simulink model "generic"  (Simulink 10.0)
settings: Solver=ode45  StartTime=0.0  StopTime=inf  RelTol=1e-3  EnableMultiTasking=on
libraries: CarMaker4SL x64, simulink x6
(part 2 of 3)

== system generic/CarMaker/IPG Vehicle/CarAndTrailer/Forces/Vehicle Forces ==
  Sync_In : Inport
  Bus Creator1 : BusCreator  Inputs=12
  Bus Creator8 : BusCreator  Inputs=16
  BusCreator1 : BusCreator  Inputs=4
  BusCreator2 : BusCreator  Inputs=9
  Demux : Demux  Outputs=16
  Demux1 : Demux  Outputs=12
  Demux2 : Demux  Outputs=13
  Forces : S-Function  FunctionName=CM_Sfun  Parameters='Forces'  SFunctionDeploymentMode=off  EnableBusSupport=off
  Terminator : Terminator
  Sync_Out : Outport
  Car.Virtual : Outport  Port=2
  Car.Aero : Outport  Port=3
  Car.Load : Outport  Port=4
  wires:
  BusCreator1/1 -> Terminator/1  "Aero IF (in)"
  Demux2/13 -> BusCreator2/9  "car Aero Trq_1 z"
  Demux2/12 -> BusCreator2/8  "car Aero Trq_1 y"
  Demux2/11 -> BusCreator2/7  "car Aero Trq_1 x"
  Demux2/10 -> BusCreator2/6  "car Aero Frc_1 z"
  Demux2/9 -> BusCreator2/5  "car Aero Frc_1 y"
  Demux2/8 -> BusCreator2/4  "car Aero Frc_1 x"
  Demux2/7 -> BusCreator2/3  "car Aero PoA_1 z"
  Demux2/6 -> BusCreator2/2  "car Aero PoA_1 y"
  Demux2/5 -> BusCreator2/1  "car Aero PoA_1 x"
  Demux2/4 -> BusCreator1/4  "car Aero tau_1"
  Demux2/3 -> BusCreator1/3  "car Aero ApproachVel_1 z"
  Demux2/2 -> BusCreator1/2  "car Aero ApproachVel_1 y"
  Demux2/1 -> BusCreator1/1  "car Aero ApproachVel_1 x"
  Demux/16 -> Bus Creator8/16  "Car Load_3 tz"
  Demux/15 -> Bus Creator8/15  "Car Load_3 ty"
  Demux/14 -> Bus Creator8/14  "Car Load_3 tx"
  Demux/13 -> Bus Creator8/13  "Car Load_3 mass"
  Demux1/12 -> Bus Creator1/12  "Car Virtual Trq_0 z"
  Demux1/11 -> Bus Creator1/11  "Car Virtual Trq_0 y"
  Demux1/10 -> Bus Creator1/10  "Car Virtual Trq_0 x"
  Demux1/9 -> Bus Creator1/9  "Car Virtual Trq_1 z"
  Demux1/8 -> Bus Creator1/8  "Car Virtual Trq_1 y"
  Demux1/7 -> Bus Creator1/7  "Car Virtual Trq_1 x"
  Demux1/6 -> Bus Creator1/6  "Car Virtual Frc_0 z"
  Demux1/5 -> Bus Creator1/5  "Car Virtual Frc_0 y"
  Demux1/4 -> Bus Creator1/4  "Car Virtual Frc_0 x"
  Sync_In/1 -> Forces/1
  Forces/1 -> Sync_Out/1
  BusCreator2/1 -> Car.Aero/1
  Demux1/1 -> Bus Creator1/1  "Car Virtual Frc_1 x"
  Demux1/2 -> Bus Creator1/2  "Car Virtual Frc_1 y"
  Demux1/3 -> Bus Creator1/3  "Car Virtual Frc_1 z"
  Forces/3 -> Demux2/1
  Forces/2 -> Demux1/1
  Bus Creator1/1 -> Car.Virtual/1
  Bus Creator8/1 -> Car.Load/1
  Demux/1 -> Bus Creator8/1  "Car Load_0 mass"
  Demux/2 -> Bus Creator8/2  "Car Load_0 tx"
  Demux/3 -> Bus Creator8/3  "Car Load_0 ty"
  Demux/4 -> Bus Creator8/4  "Car Load_0 tz"
  Demux/5 -> Bus Creator8/5  "Car Load_1 mass"
  Demux/6 -> Bus Creator8/6  "Car Load_1 tx"
  Demux/7 -> Bus Creator8/7  "Car Load_1 ty"
  Demux/8 -> Bus Creator8/8  "Car Load_1 tz"
  Demux/9 -> Bus Creator8/9  "Car Load_2 mass"
  Demux/10 -> Bus Creator8/10  "Car Load_2 tx"
  Demux/11 -> Bus Creator8/11  "Car Load_2 ty"
  Demux/12 -> Bus Creator8/12  "Car Load_2 tz"
  Forces/4 -> Demux/1

== system generic/CarMaker/IPG Vehicle/CarAndTrailer/Trailer/CreateBus Car.Hitch.FrcTrq ==
  In1 : Inport
  Bus Creator7 : BusCreator  Inputs=6
  Demux7 : Demux  Outputs=6
  Out1 : Outport
  wires:
  In1/1 -> Demux7/1
  Bus Creator7/1 -> Out1/1
  Demux7/6 -> Bus Creator7/6  "Car Hitch Trq2Car z"
  Demux7/5 -> Bus Creator7/5  "Car Hitch Trq2Car y"
  Demux7/4 -> Bus Creator7/4  "Car Hitch Trq2Car x"
  Demux7/3 -> Bus Creator7/3  "Car Hitch Frc2Car z"
  Demux7/2 -> Bus Creator7/2  "Car Hitch Frc2Car y"
  Demux7/1 -> Bus Creator7/1  "Car Hitch Frc2Car x"

== system generic/CarMaker/IPG Vehicle/CarAndTrailer/Trailer/CreateBus Vhcl.Motion ==
  In1 : Inport
  BusCreator : BusCreator  Inputs=15
  Demux : Demux  Outputs=15
  Out1 : Outport
  wires:
  Demux/15 -> BusCreator/15  "Vhcl YawAcc"
  Demux/14 -> BusCreator/14  "Vhcl YawVel"
  Demux/13 -> BusCreator/13  "Vhcl Yaw"
  Demux/12 -> BusCreator/12  "Vhcl PitchAcc"
  Demux/11 -> BusCreator/11  "Vhcl PitchVel"
  Demux/10 -> BusCreator/10  "Vhcl Pitch"
  Demux/9 -> BusCreator/9  "Vhcl RollAcc"
  Demux/8 -> BusCreator/8  "Vhcl RollVel"
  Demux/7 -> BusCreator/7  "Vhcl Roll"
  Demux/6 -> BusCreator/6  "Vhcl Hitch_Pos z"
  Demux/5 -> BusCreator/5  "Vhcl Hitch_Pos y"
  Demux/4 -> BusCreator/4  "Vhcl Hitch_Pos x"
  Demux/3 -> BusCreator/3  "Vhcl sRoad"
  Demux/2 -> BusCreator/2  "Vhcl Distance"
  Demux/1 -> BusCreator/1  "Vhcl v"
  In1/1 -> Demux/1
  BusCreator/1 -> Out1/1

== system generic/CarMaker/IPG Vehicle/CarAndTrailer/Trailer/CreateBus Vhcl.PoI ==
  In1 : Inport
  Bus Creator3 : BusCreator  Inputs=18
  Demux3 : Demux  Outputs=18
  Out1 : Outport
  wires:
  Demux3/18 -> Bus Creator3/18  "Vhcl PoI_GCS Elev"
  Demux3/17 -> Bus Creator3/17  "Vhcl PoI_GCS Lat"
  Demux3/16 -> Bus Creator3/16  "Vhcl PoI_GCS Long"
  Demux3/15 -> Bus Creator3/15  "Vhcl PoI_Acc_1 z"
  Demux3/14 -> Bus Creator3/14  "Vhcl PoI_Acc_1 y"
  Demux3/13 -> Bus Creator3/13  "Vhcl PoI_Acc_1 x"
  Demux3/12 -> Bus Creator3/12  "Vhcl PoI_Vel_1 z"
  Demux3/11 -> Bus Creator3/11  "Vhcl PoI_Vel_1 y"
  Demux3/10 -> Bus Creator3/10  "Vhcl PoI_Vel_1 x"
  Demux3/9 -> Bus Creator3/9  "Vhcl PoI_Acc z"
  Demux3/8 -> Bus Creator3/8  "Vhcl PoI_Acc y"
  Demux3/7 -> Bus Creator3/7  "Vhcl PoI_Acc x"
  Demux3/6 -> Bus Creator3/6  "Vhcl PoI_Vel z"
  Demux3/5 -> Bus Creator3/5  "Vhcl PoI_Vel y"
  Demux3/4 -> Bus Creator3/4  "Vhcl PoI_Vel x"
  Demux3/3 -> Bus Creator3/3  "Vhcl PoI_Pos z"
  Demux3/2 -> Bus Creator3/2  "Vhcl PoI_Pos y"
  In1/1 -> Demux3/1
  Bus Creator3/1 -> Out1/1
  Demux3/1 -> Bus Creator3/1  "Vhcl PoI_Pos x"

== system generic/CarMaker/IPG Vehicle/CarAndTrailer/Trailer/CreateBus Vhcl.Steering ==
  In1 : Inport
  Bus Creator3 : BusCreator  Inputs=4
  Demux : Demux
  Out1 : Outport
  wires:
  Bus Creator3/1 -> Out1/1
  Demux/1 -> Bus Creator3/1  "Vhcl Steering Ang"
  Demux/3 -> Bus Creator3/3  "Vhcl Steering AngAcc"
  Demux/2 -> Bus Creator3/2  "Vhcl Steering AngVel"
  Demux/4 -> Bus Creator3/4  "Vhcl Steering Trq"
  In1/1 -> Demux/1

== system generic/CarMaker/IPG Vehicle/CarAndTrailer/Trailer/CreateBus Vhcl.Wheel.FL ==
  In1 : Inport
  Bus Creator3 : BusCreator  Inputs=14
  Demux3 : Demux  Outputs=14
  Out1 : Outport
  wires:
  Demux3/14 -> Bus Creator3/14  "Vhcl Wheel FL Trq_WhlBearing"
  Demux3/13 -> Bus Creator3/13  "Vhcl Wheel FL Trq_T2W"
  Demux3/12 -> Bus Creator3/12  "Vhcl Wheel FL SideSlip"
  Demux3/11 -> Bus Creator3/11  "Vhcl Wheel FL LongSlip"
  Demux3/10 -> Bus Creator3/10  "Vhcl Wheel FL vBelt"
  Demux3/9 -> Bus Creator3/9  "Vhcl Wheel FL Fz"
  Demux3/8 -> Bus Creator3/8  "Vhcl Wheel FL Fy"
  Demux3/7 -> Bus Creator3/7  "Vhcl Wheel FL Fx"
  Demux3/6 -> Bus Creator3/6  "Vhcl Wheel FL r_zxy z"
  Demux3/5 -> Bus Creator3/5  "Vhcl Wheel FL r_zxy y"
  Demux3/4 -> Bus Creator3/4  "Vhcl Wheel FL r_zxy x"
  Demux3/3 -> Bus Creator3/3  "Vhcl Wheel FL t z"
  Demux3/2 -> Bus Creator3/2  "Vhcl Wheel FL t y"
  In1/1 -> Demux3/1
  Bus Creator3/1 -> Out1/1
  Demux3/1 -> Bus Creator3/1  "Vhcl Wheel FL t x"

== system generic/CarMaker/IPG Vehicle/CarAndTrailer/Trailer/CreateBus Vhcl.Wheel.FR ==
  In1 : Inport
  Bus Creator3 : BusCreator  Inputs=14
  Demux3 : Demux  Outputs=14
  Out1 : Outport
  wires:
  Demux3/14 -> Bus Creator3/14  "Vhcl Wheel FR Trq_WhlBearing"
  Demux3/13 -> Bus Creator3/13  "Vhcl Wheel FR Trq_T2W"
  Demux3/12 -> Bus Creator3/12  "Vhcl Wheel FR SideSlip"
  Demux3/11 -> Bus Creator3/11  "Vhcl Wheel FR LongSlip"
  Demux3/10 -> Bus Creator3/10  "Vhcl Wheel FR vBelt"
  Demux3/9 -> Bus Creator3/9  "Vhcl Wheel FR Fz"
  Demux3/8 -> Bus Creator3/8  "Vhcl Wheel FR Fy"
  Demux3/7 -> Bus Creator3/7  "Vhcl Wheel FR Fx"
  Demux3/6 -> Bus Creator3/6  "Vhcl Wheel FR r_zxy z"
  Demux3/5 -> Bus Creator3/5  "Vhcl Wheel FR r_zxy y"
  Demux3/4 -> Bus Creator3/4  "Vhcl Wheel FR r_zxy x"
  Demux3/3 -> Bus Creator3/3  "Vhcl Wheel FR t z"
  Demux3/2 -> Bus Creator3/2  "Vhcl Wheel FR t y"
  In1/1 -> Demux3/1
  Bus Creator3/1 -> Out1/1
  Demux3/1 -> Bus Creator3/1  "Vhcl Wheel FR t x"

== system generic/CarMaker/IPG Vehicle/CarAndTrailer/Trailer/CreateBus Vhcl.Wheel.RL ==
  In1 : Inport
  Bus Creator3 : BusCreator  Inputs=14
  Demux3 : Demux  Outputs=14
  Out1 : Outport
  wires:
  Demux3/14 -> Bus Creator3/14  "Vhcl Wheel RL Trq_WhlBearing"
  Demux3/13 -> Bus Creator3/13  "Vhcl Wheel RL Trq_T2W"
  Demux3/12 -> Bus Creator3/12  "Vhcl Wheel RL SideSlip"
  Demux3/11 -> Bus Creator3/11  "Vhcl Wheel RL LongSlip"
  Demux3/10 -> Bus Creator3/10  "Vhcl Wheel RL vBelt"
  Demux3/9 -> Bus Creator3/9  "Vhcl Wheel RL Fz"
  Demux3/8 -> Bus Creator3/8  "Vhcl Wheel RL Fy"
  Demux3/7 -> Bus Creator3/7  "Vhcl Wheel RL Fx"
  Demux3/6 -> Bus Creator3/6  "Vhcl Wheel RL r_zxy z"
  Demux3/5 -> Bus Creator3/5  "Vhcl Wheel RL r_zxy y"
  Demux3/4 -> Bus Creator3/4  "Vhcl Wheel RL r_zxy x"
  Demux3/3 -> Bus Creator3/3  "Vhcl Wheel RL t z"
  Demux3/2 -> Bus Creator3/2  "Vhcl Wheel RL t y"
  In1/1 -> Demux3/1
  Bus Creator3/1 -> Out1/1
  Demux3/1 -> Bus Creator3/1  "Vhcl Wheel RL t x"

== system generic/CarMaker/IPG Vehicle/CarAndTrailer/Trailer/CreateBus Vhcl.Wheel.RR ==
  In1 : Inport
  Bus Creator3 : BusCreator  Inputs=14
  Demux3 : Demux  Outputs=14
  Out1 : Outport
  wires:
  Demux3/14 -> Bus Creator3/14  "Vhcl Wheel RR Trq_WhlBearing"
  Demux3/13 -> Bus Creator3/13  "Vhcl Wheel RR Trq_T2W"
  Demux3/12 -> Bus Creator3/12  "Vhcl Wheel RR SideSlip"
  Demux3/11 -> Bus Creator3/11  "Vhcl Wheel RR LongSlip"
  Demux3/10 -> Bus Creator3/10  "Vhcl Wheel RR vBelt"
  Demux3/9 -> Bus Creator3/9  "Vhcl Wheel RR Fz"
  Demux3/8 -> Bus Creator3/8  "Vhcl Wheel RR Fy"
  Demux3/7 -> Bus Creator3/7  "Vhcl Wheel RR Fx"
  Demux3/6 -> Bus Creator3/6  "Vhcl Wheel RR r_zxy z"
  Demux3/5 -> Bus Creator3/5  "Vhcl Wheel RR r_zxy y"
  Demux3/4 -> Bus Creator3/4  "Vhcl Wheel RR r_zxy x"
  Demux3/3 -> Bus Creator3/3  "Vhcl Wheel RR t z"
  Demux3/2 -> Bus Creator3/2  "Vhcl Wheel RR t y"
  In1/1 -> Demux3/1
  Bus Creator3/1 -> Out1/1
  Demux3/1 -> Bus Creator3/1  "Vhcl Wheel RR t x"

== system generic/CarMaker/VehicleControl/CreateBus VhclCtrl/Braking/Front Camera ==
  Bus Selector : BusSelector  OutputSignals=MBR_TR_X,MBR_BL_Y,MBR_TR_Y,Confidence
  Camera Sensor Object : CarMaker4SL/Sensors/Camera Sensor Object  xname=Frontcamera  xstime=Inherited
      settings: SourceProductName=CarMaker4SL
  Constant1 : Constant
  Constant7 : Constant
  Data Type Conversion : DataTypeConversion  OutDataTypeStr=double
  Ground5 : Ground
  If : If  NumInputs=4  IfExpression=(u1>0&u3<0) &u4>0  ElseIfExpressions=((u1<=0.55&u1>=-0.55)|(u3<=0.55&u3>=-0.55))&u4>0,u2==0&u4>0  ShowElse=off
  If Action Subsystem : Subsystem  TreatAsAtomicUnit=on
  If Action Subsystem1 : Subsystem  TreatAsAtomicUnit=on
  If Action Subsystem2 : Subsystem  TreatAsAtomicUnit=on
  Terminator : Terminator
  While Iterator Subsystem3 : Subsystem  TreatAsAtomicUnit=on
  wires:
  Constant7/1 -> While Iterator Subsystem3/1(IC)
  Bus Selector/2 -> If Action Subsystem2/2(Inport1), If/1  "<MBR_BL_Y>"
  Bus Selector/3 -> If Action Subsystem2/3(Inport2), If/3  "<MBR_TR_Y>"
  Bus Selector/1 -> If Action Subsystem2/1(Inport), If Action Subsystem/1(Inport), If/2  "<MBR_TR_X>"
  If/3 -> If Action Subsystem1/Action
  Data Type Conversion/1 -> If/4
  If/1 -> If Action Subsystem/Action
  Camera Sensor Object/1 -> Terminator/1
  Ground5/1 -> Camera Sensor Object/1
  Constant1/1 -> Camera Sensor Object/2
  Camera Sensor Object/2 -> Bus Selector/1
  Bus Selector/4 -> Data Type Conversion/1  "<Confidence>"
  If/2 -> If Action Subsystem2/Action

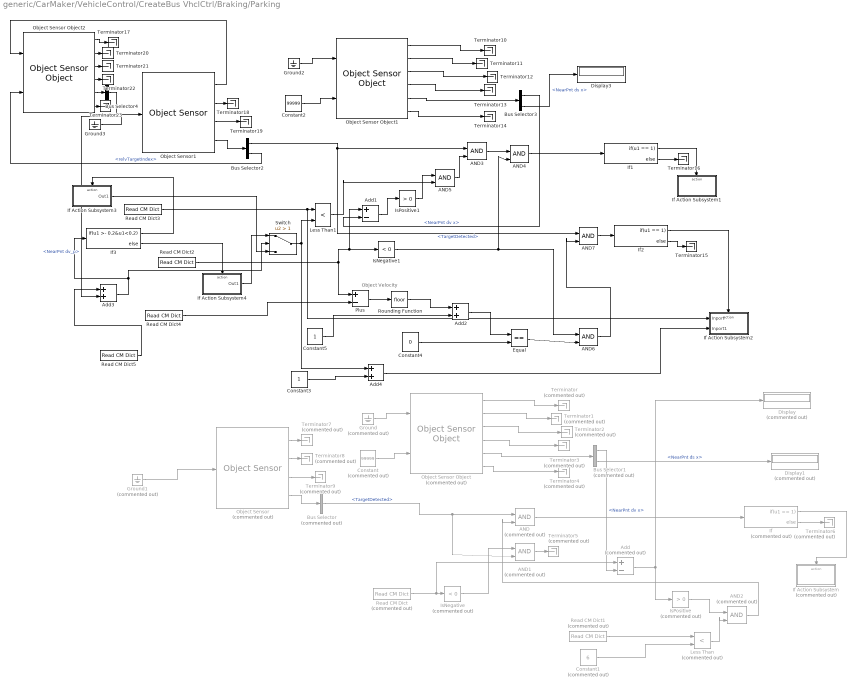
== system generic/CarMaker/VehicleControl/CreateBus VhclCtrl/Braking/Parking ==
  note: Object Velocity
  AND : Logic  Commented=on  IconShape=distinctive  AllPortsSameDT=off  OutDataTypeStr=boolean
  AND1 : Logic  Commented=on  IconShape=distinctive  AllPortsSameDT=off  OutDataTypeStr=boolean
  AND2 : Logic  Commented=on  IconShape=distinctive  AllPortsSameDT=off  OutDataTypeStr=boolean
  AND{3..7} (5 alike) : Logic  IconShape=distinctive  AllPortsSameDT=off  OutDataTypeStr=boolean
  Add : Sum  Commented=on  Inputs=+-
  Add1 : Sum  Inputs=+-
  Add2 : Sum
  Add3 : Sum
  Add4 : Sum
  Bus Selector : BusSelector  Commented=on  OutputSignals=TargetDetected
  Bus Selector1 : BusSelector  Commented=on  OutputSignals=NearPnt dv x,NearPnt ds x
  Bus Selector2 : BusSelector  OutputSignals=TargetDetected,relvTargetIndex
  Bus Selector3 : BusSelector  OutputSignals=NearPnt dv x,NearPnt ds x
  Bus Selector4 : BusSelector  OutputSignals=NearPnt dv_p
  Constant : Constant  Commented=on  Value=99999
  Constant1 : Constant  Commented=on  Value=6
  Constant2 : Constant  Value=99999
  Constant3 : Constant
  Constant4 : Constant  Value=0
  Constant5 : Constant
  Display : Display  Commented=on
  Display1 : Display  Commented=on
  Display3 : Display
  Equal : RelationalOperator  Operator===  OutDataTypeStr=boolean  RndMeth=Simplest
  Ground : Ground  Commented=on
  Ground1 : Ground  Commented=on
  Ground2 : Ground
  Ground3 : Ground
  If : If  Commented=on  IfExpression=u1 == 1
  If Action Subsystem : Subsystem  Commented=on  TreatAsAtomicUnit=on
  If Action Subsystem1 : Subsystem  TreatAsAtomicUnit=on
  If Action Subsystem2 : Subsystem  TreatAsAtomicUnit=on
  If Action Subsystem3 : Subsystem  TreatAsAtomicUnit=on
  If Action Subsystem4 : Subsystem  TreatAsAtomicUnit=on
  If1 : If  IfExpression=u1 == 1
  If2 : If  IfExpression=u1 == 1
  If3 : If  IfExpression=u1 >- 0.2&u1<0.2
  IsNegative : simulink/Logic and Bit Operations/Compare To Zero  Commented=on  relop=<  OutDataTypeStr=boolean
  IsNegative1 : simulink/Logic and Bit Operations/Compare To Zero  relop=<  OutDataTypeStr=boolean
  IsPositive : simulink/Logic and Bit Operations/Compare To Zero  Commented=on  relop=>  OutDataTypeStr=boolean
  IsPositive1 : simulink/Logic and Bit Operations/Compare To Zero  relop=>  OutDataTypeStr=boolean
  Less Than : RelationalOperator  Commented=on  Operator=<  OutDataTypeStr=boolean  RndMeth=Simplest
  Less Than1 : RelationalOperator  Operator=<  OutDataTypeStr=boolean  RndMeth=Simplest
  Object Sensor : CarMaker4SL/Sensors/Object Sensor  Commented=on  xname=RearR  xstime=Continuous
      settings: SourceProductName=CarMaker4SL
  Object Sensor Object : CarMaker4SL/Sensors/Object Sensor Object  Commented=on  xname=RearR  ximode=Observed Objects  xstime=Continuous
      settings: SourceProductName=CarMaker4SL
  Object Sensor Object1 : CarMaker4SL/Sensors/Object Sensor Object  xname=RearC  ximode=Observed Objects  xstime=Continuous
      settings: SourceProductName=CarMaker4SL
  Object Sensor Object2 : CarMaker4SL/Sensors/Object Sensor Object  xname=INPORT  ximode=Observed Objects  xstime=Continuous
      settings: SourceProductName=CarMaker4SL
  Object Sensor1 : CarMaker4SL/Sensors/Object Sensor  xname=RearC  xstime=Continuous
      settings: SourceProductName=CarMaker4SL
  Plus : Sum  Inputs=+-
  Read CM Dict : CarMaker4SL/Read CM Dict  Commented=on  xname=Car.vx  xsync=off  xstime=Continuous
  Read CM Dict1 : CarMaker4SL/Read CM Dict  Commented=on  xname=Sensor.Object.RearR.relvTgt.NearPnt.ds.x  xsync=off  xstime=Continuous
  Read CM Dict2 : CarMaker4SL/Read CM Dict  xname=Car.vx  xsync=off  xstime=Continuous
  Read CM Dict3 : CarMaker4SL/Read CM Dict  xname=Sensor.Object.RearC.relvTgt.NearPnt.ds.x  xsync=off  xstime=Continuous
  Read CM Dict4 : CarMaker4SL/Read CM Dict  xname=Sensor.Object.RearC.relvTgt.RefPnt.dv_p  xsync=off  xstime=Continuous
  Read CM Dict5 : CarMaker4SL/Read CM Dict  xname=Car.v  xsync=off  xstime=Continuous
  Rounding Function : Rounding
  Switch : Switch  Criteria=u2 > Threshold  Threshold=1
  Terminator{,1..9} (10 alike) : Terminator  Commented=on
  Terminator{10..23} (14 alike) : Terminator
  wires:
  Bus Selector3/2 -> Display3/1  "<NearPnt ds x>"
  Bus Selector2/1 -> AND3/1, AND7/1  "<TargetDetected>"
  Object Sensor Object1/1 -> Terminator10/1
  AND5/1 -> AND3/2
  Ground2/1 -> Object Sensor Object1/1
  Constant2/1 -> Object Sensor Object1/2
  Object Sensor Object1/2 -> Terminator11/1
  Object Sensor Object1/6 -> Terminator14/1
  IsPositive1/1 -> AND5/1
  Add1/1 -> IsPositive1/1
  Object Sensor Object1/4 -> Terminator13/1
  Object Sensor1/1 -> Object Sensor Object2/1
  Read CM Dict3/1 -> If Action Subsystem2/1(Inport), Less Than1/1
  Less Than1/1 -> AND5/2
  Object Sensor1/4 -> Bus Selector2/1
  If1/2 -> Terminator16/1
  Object Sensor Object1/3 -> Terminator12/1
  Object Sensor Object1/5 -> Bus Selector3/1
  Read CM Dict2/1 -> Add1/1, IsNegative1/1, Plus/1
  Bus Selector3/1 -> Add1/2  "<NearPnt dv x>"
  If1/1 -> If Action Subsystem1/Action
  Object Sensor1/2 -> Terminator18/1
  Ground3/1 -> Object Sensor1/1
  Object Sensor1/3 -> Terminator19/1
  Read CM Dict4/1 -> Plus/2
  Constant4/1 -> Equal/2
  Plus/1 -> Rounding Function/1
  Equal/1 -> AND6/2
  AND4/1 -> If1/1
  AND3/1 -> AND4/1
  IsNegative1/1 -> AND6/1, AND4/2
  Rounding Function/1 -> Add2/1
  Constant5/1 -> Add2/2
  Add2/1 -> Equal/1
  AND6/1 -> AND7/2
  AND7/1 -> If2/1
  If2/1 -> If Action Subsystem2/Action
  If2/2 -> Terminator15/1
  If/1 -> If Action Subsystem/Action
  Ground1/1 -> Object Sensor/1
  IsPositive/1 -> AND2/1
  AND/1 -> If/1
  Bus Selector1/2 -> Display1/1  "<NearPnt ds x>"
  Object Sensor/2 -> Terminator8/1
  AND2/1 -> AND/2
  Add/1 -> IsPositive/1, Display/1
  Bus Selector1/1 -> Add/2  "<NearPnt dv x>"
  Object Sensor Object/6 -> Terminator4/1
  If/2 -> Terminator6/1
  Less Than/1 -> AND2/2
  Object Sensor Object/4 -> Terminator3/1
  Constant/1 -> Object Sensor Object/2
  AND1/1 -> Terminator5/1
  Read CM Dict1/1 -> Less Than/1
  Object Sensor Object/5 -> Bus Selector1/1
  Object Sensor Object/1 -> Terminator/1
  Object Sensor/1 -> Terminator7/1
  Object Sensor/3 -> Terminator9/1
  Object Sensor Object/2 -> Terminator1/1
  Constant1/1 -> Less Than/2
  IsNegative/1 -> AND1/1
  Object Sensor Object/3 -> Terminator2/1
  Read CM Dict/1 -> Add/1, IsNegative/1
  Bus Selector/1 -> AND1/2, AND/1  "<TargetDetected>"
  Ground/1 -> Object Sensor Object/1
  Object Sensor/4 -> Bus Selector/1
  Read CM Dict5/1 -> Add3/1
  If3/1 -> If Action Subsystem3/Action
  Bus Selector2/2 -> Object Sensor Object2/2  "<relvTargetIndex>"
  Object Sensor Object2/1 -> Terminator17/1
  Object Sensor Object2/2 -> Terminator20/1
  Object Sensor Object2/3 -> Terminator21/1
  Object Sensor Object2/4 -> Terminator22/1
  Object Sensor Object2/5 -> Bus Selector4/1
  Object Sensor Object2/6 -> Terminator23/1
  Bus Selector4/1 -> Add3/2  "<NearPnt dv_p>"
  If3/2 -> If Action Subsystem4/Action
  Switch/1 -> Less Than1/2, Add4/1
  Add3/1 -> Switch/2, If3/1
  Add4/1 -> If Action Subsystem2/2(Inport1)
  Constant3/1 -> Add4/2
  If Action Subsystem4/1(Out1) -> Switch/1
  If Action Subsystem3/1(Out1) -> Switch/3

== system generic/CarMaker/VehicleControl/CreateBus VhclCtrl/Braking/Short ==
  Bus Selector : BusSelector  OutputSignals=TargetDetected
  Ground1 : Ground
  If Action Subsystem1 : Subsystem  TreatAsAtomicUnit=on
  If1 : If  IfExpression=u1 == 1
  Object Sensor : CarMaker4SL/Sensors/Object Sensor  xname=UltrasonicFront  xstime=Continuous
      settings: SourceProductName=CarMaker4SL
  Read CM Dict : CarMaker4SL/Read CM Dict  xname=Sensor.Object.UltrasonicFront.relvTgt.NearPnt.ds.x  xsync=off  xstime=Continuous
  Read CM Dict1 : CarMaker4SL/Read CM Dict  xname=Sensor.Object.UltrasonicFront.relvTgt.NearPnt.dv_p  xsync=off  xstime=Continuous
  Terminator{,2..4} (4 alike) : Terminator
  wires:
  Object Sensor/4 -> Bus Selector/1
  If1/1 -> If Action Subsystem1/Action
  Object Sensor/2 -> Terminator2/1
  If1/2 -> Terminator/1
  Read CM Dict/1 -> If Action Subsystem1/1(In1)
  Object Sensor/1 -> Terminator3/1
  Ground1/1 -> Object Sensor/1
  Read CM Dict1/1 -> If Action Subsystem1/2(In2)
  Bus Selector/1 -> If1/1  "<TargetDetected>"
  Object Sensor/3 -> Terminator4/1

== system generic/CarMaker/VehicleControl/CreateBus VhclCtrl/Braking/Subsystem6 ==
  Bus Selector1 : BusSelector  OutputSignals=nObj
  Constant1 : Constant
  Ground : Ground
  Radar Sensor : CarMaker4SL/Sensors/Radar Sensor  xname=RoadDetection  xstime=Continuous
      settings: SourceProductName=CarMaker4SL
  Terminator2 : Terminator
  While Iterator Subsystem : Subsystem  TreatAsAtomicUnit=on
  wires:
  Constant1/1 -> While Iterator Subsystem/2(Inport)
  Radar Sensor/1 -> Terminator2/1
  Bus Selector1/1 -> While Iterator Subsystem/1(Input)  "<nObj>"
  Radar Sensor/2 -> Bus Selector1/1
  Ground/1 -> Radar Sensor/1

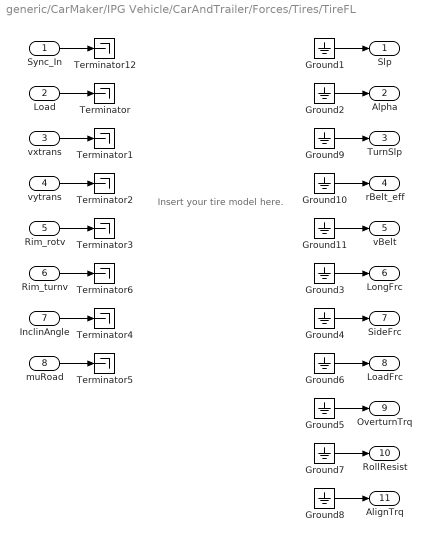
== system generic/CarMaker/IPG Vehicle/CarAndTrailer/Forces/Tires/TireFL ==
  note: Insert your tire model here.
  Sync_In : Inport
  Load : Inport  Port=2
  vxtrans : Inport  Port=3
  vytrans : Inport  Port=4
  Rim_rotv : Inport  Port=5
  Rim_turnv : Inport  Port=6
  InclinAngle : Inport  Port=7
  muRoad : Inport  Port=8
  Ground{1..11} (11 alike) : Ground
  Terminator{,1..6,12} (8 alike) : Terminator
  Slp : Outport
  Alpha : Outport  Port=2
  TurnSlp : Outport  Port=3
  rBelt_eff : Outport  Port=4
  vBelt : Outport  Port=5
  LongFrc : Outport  Port=6
  SideFrc : Outport  Port=7
  LoadFrc : Outport  Port=8
  OverturnTrq : Outport  Port=9
  RollResist : Outport  Port=10
  AlignTrq : Outport  Port=11
  wires:
  Ground11/1 -> vBelt/1
  Ground10/1 -> rBelt_eff/1
  Ground9/1 -> TurnSlp/1
  Rim_turnv/1 -> Terminator6/1
  Sync_In/1 -> Terminator12/1
  Ground2/1 -> Alpha/1
  Ground3/1 -> LongFrc/1
  Ground4/1 -> SideFrc/1
  Ground5/1 -> OverturnTrq/1
  vxtrans/1 -> Terminator1/1
  vytrans/1 -> Terminator2/1
  Rim_rotv/1 -> Terminator3/1
  InclinAngle/1 -> Terminator4/1
  muRoad/1 -> Terminator5/1
  Load/1 -> Terminator/1
  Ground1/1 -> Slp/1
  Ground6/1 -> LoadFrc/1
  Ground7/1 -> RollResist/1
  Ground8/1 -> AlignTrq/1

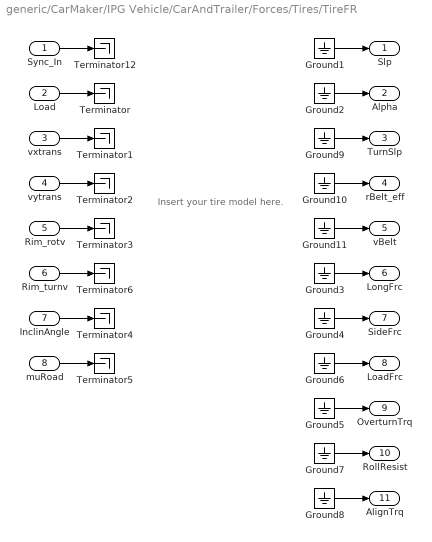
== system generic/CarMaker/IPG Vehicle/CarAndTrailer/Forces/Tires/TireFR ==
  note: Insert your tire model here.
  Sync_In : Inport
  Load : Inport  Port=2
  vxtrans : Inport  Port=3
  vytrans : Inport  Port=4
  Rim_rotv : Inport  Port=5
  Rim_turnv : Inport  Port=6
  InclinAngle : Inport  Port=7
  muRoad : Inport  Port=8
  Ground{1..11} (11 alike) : Ground
  Terminator{,1..6,12} (8 alike) : Terminator
  Slp : Outport
  Alpha : Outport  Port=2
  TurnSlp : Outport  Port=3
  rBelt_eff : Outport  Port=4
  vBelt : Outport  Port=5
  LongFrc : Outport  Port=6
  SideFrc : Outport  Port=7
  LoadFrc : Outport  Port=8
  OverturnTrq : Outport  Port=9
  RollResist : Outport  Port=10
  AlignTrq : Outport  Port=11
  wires:
  Ground11/1 -> vBelt/1
  Ground10/1 -> rBelt_eff/1
  Ground9/1 -> TurnSlp/1
  Rim_turnv/1 -> Terminator6/1
  Sync_In/1 -> Terminator12/1
  Ground2/1 -> Alpha/1
  Ground3/1 -> LongFrc/1
  Ground4/1 -> SideFrc/1
  Ground5/1 -> OverturnTrq/1
  vxtrans/1 -> Terminator1/1
  vytrans/1 -> Terminator2/1
  Rim_rotv/1 -> Terminator3/1
  InclinAngle/1 -> Terminator4/1
  muRoad/1 -> Terminator5/1
  Load/1 -> Terminator/1
  Ground1/1 -> Slp/1
  Ground6/1 -> LoadFrc/1
  Ground7/1 -> RollResist/1
  Ground8/1 -> AlignTrq/1

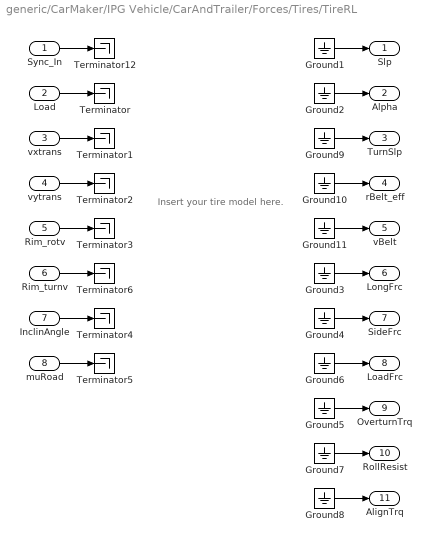
== system generic/CarMaker/IPG Vehicle/CarAndTrailer/Forces/Tires/TireRL ==
  note: Insert your tire model here.
  Sync_In : Inport
  Load : Inport  Port=2
  vxtrans : Inport  Port=3
  vytrans : Inport  Port=4
  Rim_rotv : Inport  Port=5
  Rim_turnv : Inport  Port=6
  InclinAngle : Inport  Port=7
  muRoad : Inport  Port=8
  Ground{1..11} (11 alike) : Ground
  Terminator{,1..6,12} (8 alike) : Terminator
  Slp : Outport
  Alpha : Outport  Port=2
  TurnSlp : Outport  Port=3
  rBelt_eff : Outport  Port=4
  vBelt : Outport  Port=5
  LongFrc : Outport  Port=6
  SideFrc : Outport  Port=7
  LoadFrc : Outport  Port=8
  OverturnTrq : Outport  Port=9
  RollResist : Outport  Port=10
  AlignTrq : Outport  Port=11
  wires:
  Ground11/1 -> vBelt/1
  Ground10/1 -> rBelt_eff/1
  Ground9/1 -> TurnSlp/1
  Rim_turnv/1 -> Terminator6/1
  Sync_In/1 -> Terminator12/1
  Ground2/1 -> Alpha/1
  Ground3/1 -> LongFrc/1
  Ground4/1 -> SideFrc/1
  Ground5/1 -> OverturnTrq/1
  vxtrans/1 -> Terminator1/1
  vytrans/1 -> Terminator2/1
  Rim_rotv/1 -> Terminator3/1
  InclinAngle/1 -> Terminator4/1
  muRoad/1 -> Terminator5/1
  Load/1 -> Terminator/1
  Ground1/1 -> Slp/1
  Ground6/1 -> LoadFrc/1
  Ground7/1 -> RollResist/1
  Ground8/1 -> AlignTrq/1

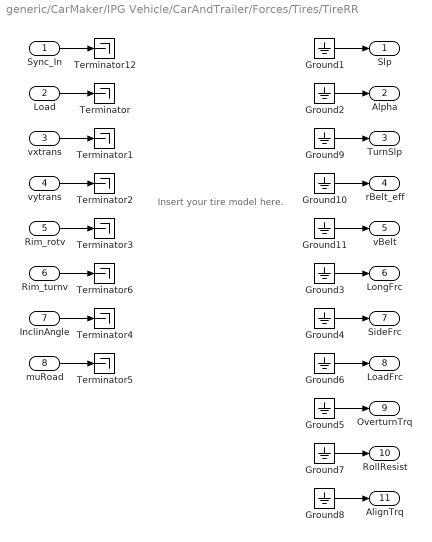
== system generic/CarMaker/IPG Vehicle/CarAndTrailer/Forces/Tires/TireRR ==
  note: Insert your tire model here.
  Sync_In : Inport
  Load : Inport  Port=2
  vxtrans : Inport  Port=3
  vytrans : Inport  Port=4
  Rim_rotv : Inport  Port=5
  Rim_turnv : Inport  Port=6
  InclinAngle : Inport  Port=7
  muRoad : Inport  Port=8
  Ground{1..11} (11 alike) : Ground
  Terminator{,1..6,12} (8 alike) : Terminator
  Slp : Outport
  Alpha : Outport  Port=2
  TurnSlp : Outport  Port=3
  rBelt_eff : Outport  Port=4
  vBelt : Outport  Port=5
  LongFrc : Outport  Port=6
  SideFrc : Outport  Port=7
  LoadFrc : Outport  Port=8
  OverturnTrq : Outport  Port=9
  RollResist : Outport  Port=10
  AlignTrq : Outport  Port=11
  wires:
  Ground11/1 -> vBelt/1
  Ground10/1 -> rBelt_eff/1
  Ground9/1 -> TurnSlp/1
  Rim_turnv/1 -> Terminator6/1
  Sync_In/1 -> Terminator12/1
  Ground2/1 -> Alpha/1
  Ground3/1 -> LongFrc/1
  Ground4/1 -> SideFrc/1
  Ground5/1 -> OverturnTrq/1
  vxtrans/1 -> Terminator1/1
  vytrans/1 -> Terminator2/1
  Rim_rotv/1 -> Terminator3/1
  InclinAngle/1 -> Terminator4/1
  muRoad/1 -> Terminator5/1
  Load/1 -> Terminator/1
  Ground1/1 -> Slp/1
  Ground6/1 -> LoadFrc/1
  Ground7/1 -> RollResist/1
  Ground8/1 -> AlignTrq/1

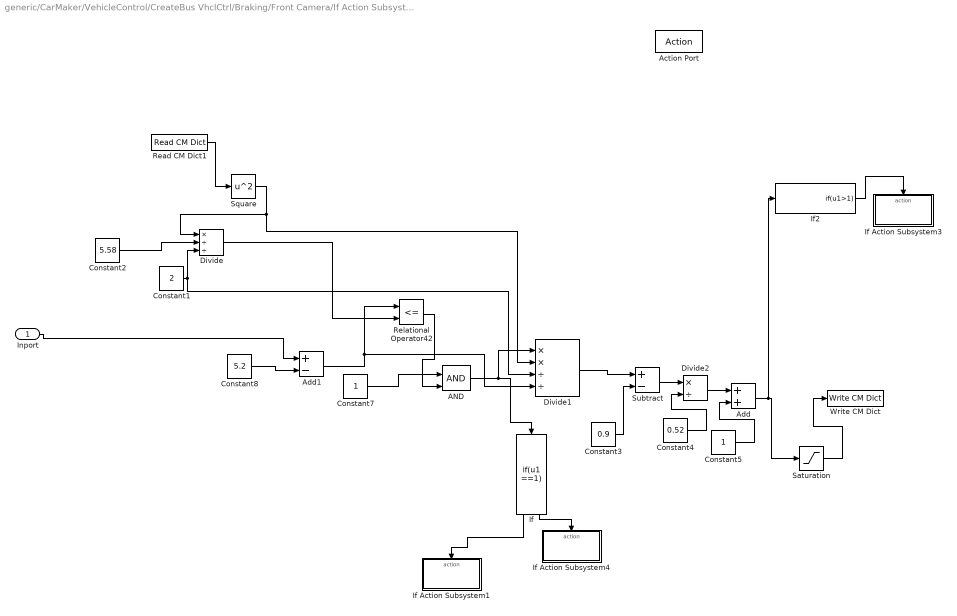
== system generic/CarMaker/VehicleControl/CreateBus VhclCtrl/Braking/Front Camera/If Action Subsystem ==
  Inport : Inport
  Action Port : ActionPort  ActionPortLabel=if((u1>0&u3<0) &u4>0)
  AND : Logic  IconShape=distinctive  AllPortsSameDT=off  OutDataTypeStr=boolean
  Add : Sum
  Add1 : Sum  Inputs=+-
  Constant1 : Constant  Value=2
  Constant2 : Constant  Value=5.58
  Constant3 : Constant  Value=0.9
  Constant4 : Constant  Value=0.52
  Constant5 : Constant
  Constant7 : Constant
  Constant8 : Constant  Value=5.2
  Divide : Product  Inputs=*//
  Divide1 : Product  Inputs=**//
  Divide2 : Product  Inputs=*/
  If : If  IfExpression=u1 ==1
  If Action Subsystem1 : Subsystem  TreatAsAtomicUnit=on
  If Action Subsystem3 : Subsystem  TreatAsAtomicUnit=on
  If Action Subsystem4 : Subsystem  TreatAsAtomicUnit=on
  If2 : If  IfExpression=u1>1  ShowElse=off
  Read CM Dict1 : CarMaker4SL/Read CM Dict  xname=Car.vx  xsync=off  xstime=Inherited
  Relational Operator42 : RelationalOperator  Operator=<=  OutDataTypeStr=boolean  RndMeth=Simplest
  Saturation : Saturate  UpperLimit=1  LowerLimit=0
  Square : Math  Operator=square  SaturateOnIntegerOverflow=on
  Subtract : Sum  Inputs=+-
  Write CM Dict : CarMaker4SL/Write CM Dict  xname=VC.Brake  xsync=off
  wires:
  AND/1 -> If/1, Divide1/1
  If/2 -> If Action Subsystem4/Action
  Subtract/1 -> Divide2/1
  Add1/1 -> Divide1/4, Relational Operator42/1
  Square/1 -> Divide1/2, Divide/1
  Saturation/1 -> Write CM Dict/1
  Constant4/1 -> Divide2/2
  Constant7/1 -> AND/1
  Constant5/1 -> Add/2
  Constant2/1 -> Divide/2
  Constant8/1 -> Add1/2
  Constant3/1 -> Subtract/2
  Divide1/1 -> Subtract/1
  If/1 -> If Action Subsystem1/Action
  Constant1/1 -> Divide/3, Divide1/3
  Inport/1 -> Add1/1
  Divide2/1 -> Add/1
  Read CM Dict1/1 -> Square/1
  Divide/1 -> Relational Operator42/2
  Relational Operator42/1 -> AND/2
  Add/1 -> If2/1, Saturation/1
  If2/1 -> If Action Subsystem3/Action

== system generic/CarMaker/VehicleControl/CreateBus VhclCtrl/Braking/Front Camera/If Action Subsystem1 ==
  Action Port : ActionPort  ActionPortLabel=elseif(u2==0&u4>0)
  Constant : Constant
  Constant1 : Constant
  Write CM Dict : CarMaker4SL/Write CM Dict  xname=VC.Brake  xsync=off
  Write CM Dict1 : CarMaker4SL/Write CM Dict  xname=VC.Gas  xsync=off
  wires:
  Constant/1 -> Write CM Dict/1
  Constant1/1 -> Write CM Dict1/1

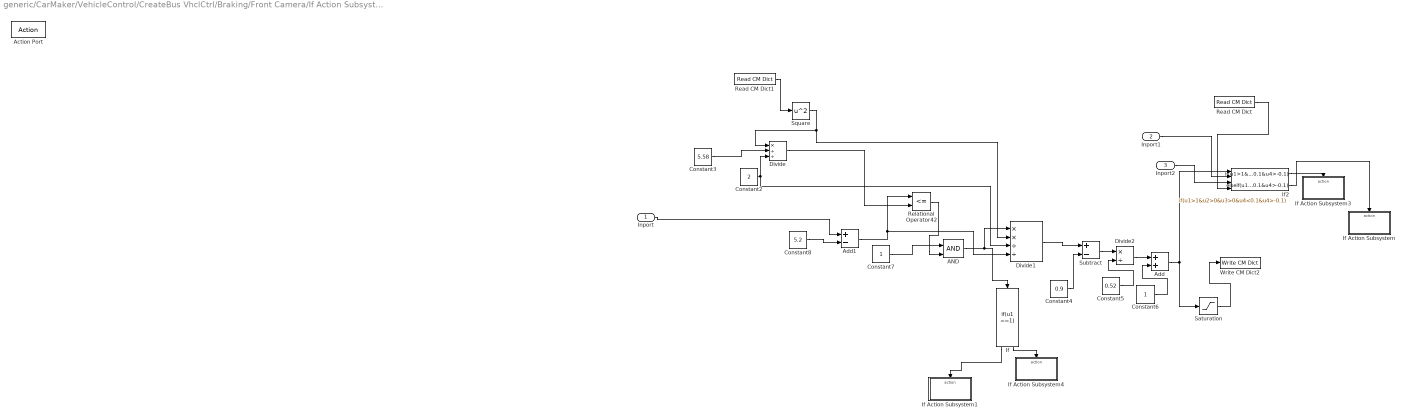
== system generic/CarMaker/VehicleControl/CreateBus VhclCtrl/Braking/Front Camera/If Action Subsystem2 ==
  Inport : Inport
  Inport1 : Inport  Port=2
  Inport2 : Inport  Port=3
  Action Port : ActionPort  ActionPortLabel=elseif(((u1<=0.55&u1>=-0.55)|(u3<=0.55&u3>=-0.55))&u4>0)
  AND : Logic  IconShape=distinctive  AllPortsSameDT=off  OutDataTypeStr=boolean
  Add : Sum
  Add1 : Sum  Inputs=+-
  Constant2 : Constant  Value=2
  Constant3 : Constant  Value=5.58
  Constant4 : Constant  Value=0.9
  Constant5 : Constant  Value=0.52
  Constant6 : Constant
  Constant7 : Constant
  Constant8 : Constant  Value=5.2
  Divide : Product  Inputs=*//
  Divide1 : Product  Inputs=**//
  Divide2 : Product  Inputs=*/
  If : If  IfExpression=u1 ==1
  If Action Subsystem : Subsystem  TreatAsAtomicUnit=on
  If Action Subsystem1 : Subsystem  TreatAsAtomicUnit=on
  If Action Subsystem3 : Subsystem  TreatAsAtomicUnit=on
  If Action Subsystem4 : Subsystem  TreatAsAtomicUnit=on
  If2 : If  NumInputs=4  IfExpression=u1>1&u2>0&u3>0&u4<0.1&u4>-0.1  ElseIfExpressions=u1>1&u2<0&u3<0&u4<0.1&u4>-0.1  ShowElse=off
  Read CM Dict : CarMaker4SL/Read CM Dict  xname=DM.Steer.Ang  xsync=off  xstime=Inherited
  Read CM Dict1 : CarMaker4SL/Read CM Dict  xname=Car.vx  xsync=off  xstime=Inherited
  Relational Operator42 : RelationalOperator  Operator=<=  OutDataTypeStr=boolean  RndMeth=Simplest
  Saturation : Saturate  UpperLimit=1  LowerLimit=0
  Square : Math  Operator=square  SaturateOnIntegerOverflow=on
  Subtract : Sum  Inputs=+-
  Write CM Dict2 : CarMaker4SL/Write CM Dict  xname=VC.Brake  xsync=off
  wires:
  Subtract/1 -> Divide2/1
  Divide/1 -> Relational Operator42/2
  Relational Operator42/1 -> AND/2
  Constant8/1 -> Add1/2
  Read CM Dict1/1 -> Square/1
  Saturation/1 -> Write CM Dict2/1
  Square/1 -> Divide1/2, Divide/1
  Divide2/1 -> Add/1
  Inport/1 -> Add1/1
  Constant5/1 -> Divide2/2
  Constant7/1 -> AND/1
  Constant2/1 -> Divide/3, Divide1/3
  Constant3/1 -> Divide/2
  If/1 -> If Action Subsystem1/Action
  Divide1/1 -> Subtract/1
  AND/1 -> If/1, Divide1/1
  Constant6/1 -> Add/2
  Add1/1 -> Divide1/4, Relational Operator42/1
  Constant4/1 -> Subtract/2
  If/2 -> If Action Subsystem4/Action
  Read CM Dict/1 -> If2/4
  Add/1 -> If2/1, Saturation/1
  If2/2 -> If Action Subsystem/Action
  If2/1 -> If Action Subsystem3/Action
  Inport1/1 -> If2/2
  Inport2/1 -> If2/3

== system generic/CarMaker/VehicleControl/CreateBus VhclCtrl/Braking/Front Camera/While Iterator Subsystem3 ==
  IC : Inport
  Bus Selector : BusSelector  OutputSignals=MBR_TR_X,MBR_BL_Y,MBR_TR_Y,Confidence
  Camera Sensor Object : CarMaker4SL/Sensors/Camera Sensor Object  xname=Frontcamera  xstime=Inherited
      settings: SourceProductName=CarMaker4SL
  Constant : Constant
  Constant1 : Constant
  Constant2 : Constant  Value=0
  Data Type Conversion : DataTypeConversion  OutDataTypeStr=double
  Ground5 : Ground
  If : If  NumInputs=4  IfExpression=(u1>0&u3<0) &u4>0  ElseIfExpressions=((u1<=0.55&u1>=-0.55)|(u3<=0.55&u3>=-0.55))&u4>0,u2==0&u4>0  ShowElse=off
  If Action Subsystem : Subsystem  TreatAsAtomicUnit=on
  If Action Subsystem1 : Subsystem  TreatAsAtomicUnit=on
  If Action Subsystem2 : Subsystem  TreatAsAtomicUnit=on
  Subtract : Sum  Inputs=+-
  Terminator : Terminator
  While Iterator : WhileIterator  MaxIters=4  ShowIterationPort=on
  wires:
  IC/1 -> While Iterator/2
  Ground5/1 -> Camera Sensor Object/1
  Camera Sensor Object/2 -> Bus Selector/1
  Camera Sensor Object/1 -> Terminator/1
  If/1 -> If Action Subsystem/Action
  Bus Selector/1 -> If Action Subsystem2/1(Inport), If Action Subsystem/1(Inport), If/2  "<MBR_TR_X>"
  Constant1/1 -> Subtract/2
  Constant/1 -> While Iterator/1
  Bus Selector/4 -> Data Type Conversion/1  "<Confidence>"
  Data Type Conversion/1 -> If/4
  If/2 -> If Action Subsystem2/Action
  Bus Selector/2 -> If/1  "<MBR_BL_Y>"
  Bus Selector/3 -> If/3  "<MBR_TR_Y>"
  While Iterator/1 -> Subtract/1
  If/3 -> If Action Subsystem1/Action
  Constant2/1 -> Camera Sensor Object/2

== system generic/CarMaker/VehicleControl/CreateBus VhclCtrl/Braking/Parking/If Action Subsystem ==
  Action Port : ActionPort
  Constant : Constant  Value=0
  Constant1 : Constant
  Write CM Dict : CarMaker4SL/Write CM Dict  xname=VC.Gas  xsync=off
  Write CM Dict1 : CarMaker4SL/Write CM Dict  xname=VC.Brake  xsync=off
  wires:
  Constant/1 -> Write CM Dict/1
  Constant1/1 -> Write CM Dict1/1

== system generic/CarMaker/VehicleControl/CreateBus VhclCtrl/Braking/Parking/If Action Subsystem1 ==
  Action Port : ActionPort  ActionPortLabel=if(u1 == 1)
  Constant : Constant  Value=0
  Constant1 : Constant
  Write CM Dict : CarMaker4SL/Write CM Dict  xname=VC.Gas  xsync=off
  Write CM Dict1 : CarMaker4SL/Write CM Dict  xname=VC.Brake  xsync=off
  wires:
  Constant/1 -> Write CM Dict/1
  Constant1/1 -> Write CM Dict1/1

== system generic/CarMaker/VehicleControl/CreateBus VhclCtrl/Braking/Parking/If Action Subsystem2 ==
  Inport : Inport
  Inport1 : Inport  Port=2
  Action Port : ActionPort  ActionPortLabel=if(u1 == 1)
  Constant1 : Constant  Value=1.4
  If : If  NumInputs=2  IfExpression=u1 ==1 &u2~=1  ElseIfExpressions=u2==1 &u1==1
  If Action Subsystem : Subsystem  TreatAsAtomicUnit=on
  If Action Subsystem1 : Subsystem  TreatAsAtomicUnit=on
  Less Than : RelationalOperator  Operator=<  OutDataTypeStr=boolean  RndMeth=Simplest
  Less Than1 : RelationalOperator  Operator=<  OutDataTypeStr=boolean  RndMeth=Simplest
  Terminator : Terminator
  wires:
  Inport/1 -> Less Than1/1, Less Than/1
  Inport1/1 -> Less Than/2
  Less Than/1 -> If/1
  If/3 -> Terminator/1
  If/1 -> If Action Subsystem/Action
  Constant1/1 -> Less Than1/2
  If/2 -> If Action Subsystem1/Action
  Less Than1/1 -> If/2

== system generic/CarMaker/VehicleControl/CreateBus VhclCtrl/Braking/Parking/If Action Subsystem3 ==
  Action Port : ActionPort  ActionPortLabel=if(u1 >- 0.2&u1<0.2)
  Constant : Constant
  Out1 : Outport
  wires:
  Constant/1 -> Out1/1

== system generic/CarMaker/VehicleControl/CreateBus VhclCtrl/Braking/Parking/If Action Subsystem4 ==
  Action Port : ActionPort  ActionPortLabel=else
  Constant : Constant  Value=5
  Out1 : Outport
  wires:
  Constant/1 -> Out1/1

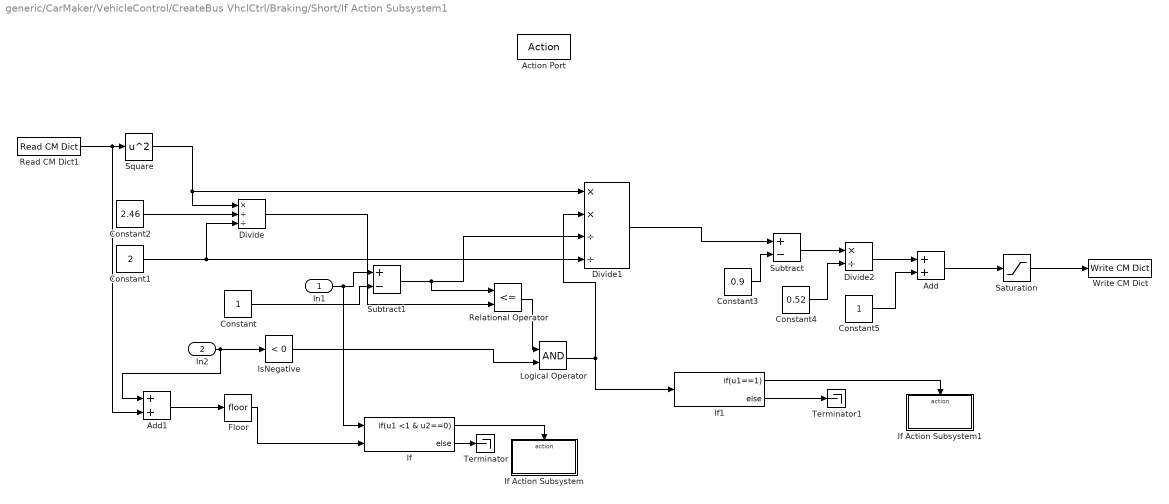
== system generic/CarMaker/VehicleControl/CreateBus VhclCtrl/Braking/Short/If Action Subsystem1 ==
  In1 : Inport
  In2 : Inport  Port=2
  Action Port : ActionPort  ActionPortLabel=if(u1 == 1)
  Add : Sum
  Add1 : Sum
  Constant : Constant
  Constant1 : Constant  Value=2
  Constant2 : Constant  Value=2.46  VectorParams1D=off
  Constant3 : Constant  Value=0.9
  Constant4 : Constant  Value=0.52
  Constant5 : Constant
  Divide : Product  Inputs=*//
  Divide1 : Product  Inputs=**//
  Divide2 : Product  Inputs=*/
  Floor : Rounding
  If : If  NumInputs=2  IfExpression=u1 <1 & u2==0
  If Action Subsystem : Subsystem  TreatAsAtomicUnit=on
  If Action Subsystem1 : Subsystem  TreatAsAtomicUnit=on
  If1 : If  IfExpression=u1==1
  IsNegative : simulink/Logic and Bit Operations/Compare To Zero  relop=<  OutDataTypeStr=boolean
  Logical Operator : Logic  AllPortsSameDT=off  OutDataTypeStr=boolean
  Read CM Dict1 : CarMaker4SL/Read CM Dict  xname=Car.vx  xsync=off  xstime=Continuous
  Relational Operator : RelationalOperator  Operator=<=  OutDataTypeStr=boolean  RndMeth=Simplest
  Saturation : Saturate  UpperLimit=1  LowerLimit=0
  Square : Math  Operator=square  SaturateOnIntegerOverflow=on
  Subtract : Sum  Inputs=+-
  Subtract1 : Sum  Inputs=+-
  Terminator : Terminator
  Terminator1 : Terminator
  Write CM Dict : CarMaker4SL/Write CM Dict  xname=VC.Brake  xsync=off
  wires:
  Add/1 -> Saturation/1
  Constant3/1 -> Subtract/2
  Relational Operator/1 -> Logical Operator/1
  IsNegative/1 -> Logical Operator/2
  Divide2/1 -> Add/1
  Divide1/1 -> Subtract/1
  Subtract/1 -> Divide2/1
  Read CM Dict1/1 -> Add1/2, Square/1
  Constant1/1 -> Divide/3, Divide1/4
  Constant4/1 -> Divide2/2
  Logical Operator/1 -> Divide1/2, If1/1
  In1/1 -> If/1, Subtract1/1
  If1/2 -> Terminator1/1
  Divide/1 -> Relational Operator/2
  Saturation/1 -> Write CM Dict/1
  Square/1 -> Divide1/1, Divide/1
  Constant2/1 -> Divide/2
  Constant5/1 -> Add/2
  If1/1 -> If Action Subsystem1/Action
  In2/1 -> Add1/1, IsNegative/1
  Constant/1 -> Subtract1/2
  Subtract1/1 -> Relational Operator/1, Divide1/3
  If/2 -> Terminator/1
  If/1 -> If Action Subsystem/Action
  Add1/1 -> Floor/1
  Floor/1 -> If/2

== system generic/CarMaker/VehicleControl/CreateBus VhclCtrl/Braking/Subsystem6/While Iterator Subsystem ==
  Input : Inport
  Inport : Inport  Port=2
  Bus Selector : BusSelector  OutputSignals=DistY,DistX,VrelX,DistZ
  Constant1 : Constant
  Ground1 : Ground
  If : If  NumInputs=4  IfExpression=u1<0.4&u1>-0.4&u4~=0&u3<0.3&u3>-0.3&u1<1  ShowElse=off
  If Action Subsystem1 : Subsystem  TreatAsAtomicUnit=on
  Radar Sensor Object : CarMaker4SL/Sensors/Radar Sensor Object  xname=RoadDetection  ximode=Observed Objects  xstime=Inherited
      settings: SourceProductName=CarMaker4SL
  Read CM Dict1 : CarMaker4SL/Read CM Dict  xname=Car.vx  xsync=off  xstime=Inherited
  Relational Operator : RelationalOperator  OutDataTypeStr=boolean  RndMeth=Simplest
  Subtract : Sum  Inputs=+-
  Terminator : Terminator
  VxO : Sum
  While Iterator : WhileIterator  MaxIters=100  ResetStates=reset  ShowIterationPort=on
  wires:
  Inport/1 -> While Iterator/2
  Ground1/1 -> Radar Sensor Object/1
  Radar Sensor Object/1 -> Terminator/1
  While Iterator/1 -> Relational Operator/2, Subtract/1
  Bus Selector/1 -> If/1  "<DistY>"
  Radar Sensor Object/2 -> Bus Selector/1
  Subtract/1 -> Radar Sensor Object/2
  Bus Selector/2 -> If Action Subsystem1/1(Inport), If/2  "<DistX>"
  Constant1/1 -> Subtract/2
  Read CM Dict1/1 -> VxO/1
  VxO/1 -> If/3
  Input/1 -> Relational Operator/1
  Relational Operator/1 -> While Iterator/1
  If/1 -> If Action Subsystem1/Action
  Bus Selector/3 -> VxO/2  "<VrelX>"
  Bus Selector/4 -> If/4  "<DistZ>"

== system generic/CarMaker/VehicleControl/CreateBus VhclCtrl/Braking/Front Camera/If Action Subsystem/If Action Subsystem1 ==
  Action Port : ActionPort  ActionPortLabel=if(u1 ==1)
  Constant : Constant  Value=0
  Write CM Dict1 : CarMaker4SL/Write CM Dict  xname=VC.Gas  xsync=off
  wires:
  Constant/1 -> Write CM Dict1/1

== system generic/CarMaker/VehicleControl/CreateBus VhclCtrl/Braking/Front Camera/If Action Subsystem/If Action Subsystem3 ==
  Action Port : ActionPort  ActionPortLabel=if(u1>1)
  Constant : Constant  Commented=on  Value=30
  Constant1 : Constant  Commented=on  Value=-3
  Write CM Dict : CarMaker4SL/Write CM Dict  Commented=on  xname=VC.Steer.AngAcc  xsync=off
  Write CM Dict1 : CarMaker4SL/Write CM Dict  Commented=on  xname=VC.Steer.Ang  xsync=off
  wires:
  Constant/1 -> Write CM Dict/1
  Constant1/1 -> Write CM Dict1/1

== system generic/CarMaker/VehicleControl/CreateBus VhclCtrl/Braking/Front Camera/If Action Subsystem/If Action Subsystem4 ==
  Action Port : ActionPort  ActionPortLabel=else

== system generic/CarMaker/VehicleControl/CreateBus VhclCtrl/Braking/Front Camera/If Action Subsystem2/If Action Subsystem ==
  Action Port : ActionPort  ActionPortLabel=elseif(u1>1&u2<0&u3<0&u4<0.1&u4>-0.1)
  Constant : Constant  Value=30
  Constant1 : Constant  Value=2
  Write CM Dict : CarMaker4SL/Write CM Dict  xname=VC.Steer.AngAcc  xsync=off
  Write CM Dict1 : CarMaker4SL/Write CM Dict  xname=VC.Steer.Ang  xsync=off
  wires:
  Constant1/1 -> Write CM Dict1/1
  Constant/1 -> Write CM Dict/1

== system generic/CarMaker/VehicleControl/CreateBus VhclCtrl/Braking/Front Camera/If Action Subsystem2/If Action Subsystem1 ==
  Action Port : ActionPort  ActionPortLabel=if(u1 ==1)
  Constant : Constant  Value=0
  Write CM Dict1 : CarMaker4SL/Write CM Dict  xname=VC.Gas  xsync=off
  wires:
  Constant/1 -> Write CM Dict1/1

== system generic/CarMaker/VehicleControl/CreateBus VhclCtrl/Braking/Front Camera/If Action Subsystem2/If Action Subsystem3 ==
  Action Port : ActionPort  ActionPortLabel=if(u1>1&u2>0&u3>0&u4<0.1&u4>-0.1)
  Constant : Constant  Value=-30
  Constant1 : Constant  Value=-2
  Write CM Dict : CarMaker4SL/Write CM Dict  xname=VC.Steer.AngAcc  xsync=off
  Write CM Dict1 : CarMaker4SL/Write CM Dict  xname=VC.Steer.Ang  xsync=off
  wires:
  Constant/1 -> Write CM Dict/1
  Constant1/1 -> Write CM Dict1/1

== system generic/CarMaker/VehicleControl/CreateBus VhclCtrl/Braking/Front Camera/If Action Subsystem2/If Action Subsystem4 ==
  Action Port : ActionPort  ActionPortLabel=else

== system generic/CarMaker/VehicleControl/CreateBus VhclCtrl/Braking/Front Camera/While Iterator Subsystem3/If Action Subsystem ==
  Inport : Inport
  Action Port : ActionPort  ActionPortLabel=if((u1>0&u3<0) &u4>0)
  AND : Logic  IconShape=distinctive  AllPortsSameDT=off  OutDataTypeStr=boolean
  Add : Sum
  Add1 : Sum  Inputs=+-
  Constant1 : Constant  Value=2
  Constant2 : Constant  Value=5.58
  Constant3 : Constant  Value=0.9
  Constant4 : Constant  Value=0.52
  Constant5 : Constant
  Constant7 : Constant
  Constant8 : Constant  Value=5.2
  Divide : Product  Inputs=*//
  Divide1 : Product  Inputs=**//
  Divide2 : Product  Inputs=*/
  If : If  IfExpression=u1 ==1
  If Action Subsystem1 : Subsystem  TreatAsAtomicUnit=on
  If Action Subsystem2 : Subsystem  TreatAsAtomicUnit=on
  If Action Subsystem4 : Subsystem  TreatAsAtomicUnit=on
  If1 : If  IfExpression=u1>1  ShowElse=off
  Read CM Dict1 : CarMaker4SL/Read CM Dict  xname=Car.vx  xsync=off  xstime=Inherited
  Relational Operator42 : RelationalOperator  Operator=<=  OutDataTypeStr=boolean  RndMeth=Simplest
  Saturation : Saturate  UpperLimit=1  LowerLimit=0
  Square : Math  Operator=square  SaturateOnIntegerOverflow=on
  Subtract : Sum  Inputs=+-
  Write CM Dict : CarMaker4SL/Write CM Dict  xname=VC.Brake  xsync=off
  wires:
  AND/1 -> If/1, Divide1/1
  If/2 -> If Action Subsystem4/Action
  Subtract/1 -> Divide2/1
  Add1/1 -> Divide1/4, Relational Operator42/1
  If1/1 -> If Action Subsystem2/Action
  Square/1 -> Divide1/2, Divide/1
  Add/1 -> If1/1, Saturation/1
  Saturation/1 -> Write CM Dict/1
  Constant4/1 -> Divide2/2
  Constant7/1 -> AND/1
  Constant5/1 -> Add/2
  Constant2/1 -> Divide/2
  Constant8/1 -> Add1/2
  Constant3/1 -> Subtract/2
  Divide1/1 -> Subtract/1
  If/1 -> If Action Subsystem1/Action
  Constant1/1 -> Divide/3, Divide1/3
  Inport/1 -> Add1/1
  Divide2/1 -> Add/1
  Read CM Dict1/1 -> Square/1
  Divide/1 -> Relational Operator42/2
  Relational Operator42/1 -> AND/2

== system generic/CarMaker/VehicleControl/CreateBus VhclCtrl/Braking/Front Camera/While Iterator Subsystem3/If Action Subsystem1 ==
  Action Port : ActionPort  ActionPortLabel=elseif(u2==0&u4>0)
  Constant : Constant
  Constant1 : Constant
  Write CM Dict : CarMaker4SL/Write CM Dict  xname=VC.Brake  xsync=off
  Write CM Dict1 : CarMaker4SL/Write CM Dict  xname=VC.Gas  xsync=off
  wires:
  Constant/1 -> Write CM Dict/1
  Constant1/1 -> Write CM Dict1/1

== system generic/CarMaker/VehicleControl/CreateBus VhclCtrl/Braking/Front Camera/While Iterator Subsystem3/If Action Subsystem2 ==
  Inport : Inport
  Action Port : ActionPort  ActionPortLabel=elseif(((u1<=0.55&u1>=-0.55)|(u3<=0.55&u3>=-0.55))&u4>0)
  AND : Logic  IconShape=distinctive  AllPortsSameDT=off  OutDataTypeStr=boolean
  Add : Sum
  Add1 : Sum  Inputs=+-
  Constant2 : Constant  Value=2
  Constant3 : Constant  Value=5.58
  Constant4 : Constant  Value=0.9
  Constant5 : Constant  Value=0.52
  Constant6 : Constant
  Constant7 : Constant
  Constant8 : Constant  Value=5.2
  Divide : Product  Inputs=*//
  Divide1 : Product  Inputs=**//
  Divide2 : Product  Inputs=*/
  If : If  IfExpression=u1 ==1
  If Action Subsystem1 : Subsystem  TreatAsAtomicUnit=on
  If Action Subsystem2 : Subsystem  TreatAsAtomicUnit=on
  If Action Subsystem4 : Subsystem  TreatAsAtomicUnit=on
  If1 : If  IfExpression=u1>1  ShowElse=off
  Read CM Dict1 : CarMaker4SL/Read CM Dict  xname=Car.vx  xsync=off  xstime=Inherited
  Relational Operator42 : RelationalOperator  Operator=<=  OutDataTypeStr=boolean  RndMeth=Simplest
  Saturation : Saturate  UpperLimit=1  LowerLimit=0
  Square : Math  Operator=square  SaturateOnIntegerOverflow=on
  Subtract : Sum  Inputs=+-
  Write CM Dict2 : CarMaker4SL/Write CM Dict  xname=VC.Brake  xsync=off
  wires:
  Subtract/1 -> Divide2/1
  Divide/1 -> Relational Operator42/2
  Relational Operator42/1 -> AND/2
  Constant8/1 -> Add1/2
  Read CM Dict1/1 -> Square/1
  If1/1 -> If Action Subsystem2/Action
  Saturation/1 -> Write CM Dict2/1
  Square/1 -> Divide1/2, Divide/1
  Divide2/1 -> Add/1
  Inport/1 -> Add1/1
  Constant5/1 -> Divide2/2
  Constant7/1 -> AND/1
  Constant2/1 -> Divide/3, Divide1/3
  Constant3/1 -> Divide/2
  If/1 -> If Action Subsystem1/Action
  Divide1/1 -> Subtract/1
  AND/1 -> If/1, Divide1/1
  Constant6/1 -> Add/2
  Add1/1 -> Divide1/4, Relational Operator42/1
  Constant4/1 -> Subtract/2
  If/2 -> If Action Subsystem4/Action
  Add/1 -> If1/1, Saturation/1

== system generic/CarMaker/VehicleControl/CreateBus VhclCtrl/Braking/Parking/If Action Subsystem2/If Action Subsystem ==
  Action Port : ActionPort  ActionPortLabel=if(u1 ==1 &u2~=1)
  Constant : Constant  Value=0.1
  Write CM Dict : CarMaker4SL/Write CM Dict  xname=VC.Brake  xsync=off
  wires:
  Constant/1 -> Write CM Dict/1

== system generic/CarMaker/VehicleControl/CreateBus VhclCtrl/Braking/Parking/If Action Subsystem2/If Action Subsystem1 ==
  Action Port : ActionPort  ActionPortLabel=elseif(u2==1 &u1==1)
  Constant : Constant  Value=0
  Constant1 : Constant
  Write CM Dict : CarMaker4SL/Write CM Dict  xname=VC.Gas  xsync=off
  Write CM Dict1 : CarMaker4SL/Write CM Dict  xname=VC.Brake  xsync=off
  wires:
  Constant/1 -> Write CM Dict/1
  Constant1/1 -> Write CM Dict1/1

== system generic/CarMaker/VehicleControl/CreateBus VhclCtrl/Braking/Short/If Action Subsystem1/If Action Subsystem ==
  Action Port : ActionPort  ActionPortLabel=if(u1 <1 & u2==0)
  Constant : Constant
  Constant1 : Constant  Value=0
  Write CM Dict : CarMaker4SL/Write CM Dict  xname=VC.Brake  xsync=off
  Write CM Dict1 : CarMaker4SL/Write CM Dict  xname=VC.Gas  xsync=off
  wires:
  Constant/1 -> Write CM Dict/1
  Constant1/1 -> Write CM Dict1/1

== system generic/CarMaker/VehicleControl/CreateBus VhclCtrl/Braking/Short/If Action Subsystem1/If Action Subsystem1 ==
  Action Port : ActionPort  ActionPortLabel=if(u1==1)
  Constant : Constant  Value=0
  Write CM Dict2 : CarMaker4SL/Write CM Dict  xname=VC.Gas  xsync=off
  wires:
  Constant/1 -> Write CM Dict2/1

== system generic/CarMaker/VehicleControl/CreateBus VhclCtrl/Braking/Subsystem6/While Iterator Subsystem/If Action Subsystem1 ==
  Inport : Inport
  Action Port : ActionPort  ActionPortLabel=if(u1<0.4&u1>-0.4&u4~=0&u3<0.3&u3>-0.3&u1<1)
  AND : Logic  IconShape=distinctive  AllPortsSameDT=off  OutDataTypeStr=boolean
  Add : Sum
  Add1 : Sum  Inputs=+-
  Constant1 : Constant  Value=2
  Constant2 : Constant  Value=2.56
  Constant3 : Constant  Value=0.9
  Constant4 : Constant  Value=0.52
  Constant5 : Constant
  Constant7 : Constant
  Constant8 : Constant  Value=0.5
  Divide : Product  Inputs=*//
  Divide1 : Product  Inputs=**//
  Divide2 : Product  Inputs=*/
  If : If  IfExpression=u1 ==1
  If Action Subsystem1 : Subsystem  TreatAsAtomicUnit=on
  If Action Subsystem2 : Subsystem  TreatAsAtomicUnit=on
  If Action Subsystem4 : Subsystem  TreatAsAtomicUnit=on
  If1 : If  IfExpression=u1>1  ShowElse=off
  Read CM Dict1 : CarMaker4SL/Read CM Dict  xname=Car.vx  xsync=off  xstime=Inherited
  Relational Operator43 : RelationalOperator  Operator=<=  OutDataTypeStr=boolean  RndMeth=Simplest
  Saturation : Saturate  UpperLimit=1  LowerLimit=0
  Square : Math  Operator=square  SaturateOnIntegerOverflow=on
  Subtract : Sum  Inputs=+-
  Write CM Dict : CarMaker4SL/Write CM Dict  xname=VC.Brake  xsync=off
  wires:
  Constant2/1 -> Divide/2
  Constant1/1 -> Divide/3, Divide1/3
  Divide2/1 -> Add/1
  Constant4/1 -> Divide2/2
  Constant7/1 -> AND/1
  Inport/1 -> Add1/1
  If1/1 -> If Action Subsystem2/Action
  Read CM Dict1/1 -> Square/1
  Constant8/1 -> Add1/2
  Saturation/1 -> Write CM Dict/1
  Square/1 -> Divide1/2, Divide/1
  Relational Operator43/1 -> AND/2
  Divide/1 -> Relational Operator43/2
  Subtract/1 -> Divide2/1
  AND/1 -> If/1, Divide1/1
  Constant5/1 -> Add/2
  Add1/1 -> Divide1/4, Relational Operator43/1
  Divide1/1 -> Subtract/1
  If/1 -> If Action Subsystem1/Action
  Constant3/1 -> Subtract/2
  Add/1 -> If1/1, Saturation/1
  If/2 -> If Action Subsystem4/Action

== system generic/CarMaker/VehicleControl/CreateBus VhclCtrl/Braking/Front Camera/While Iterator Subsystem3/If Action Subsystem/If Action Subsystem1 ==
  Action Port : ActionPort  ActionPortLabel=if(u1 ==1)
  Constant : Constant  Value=0
  Write CM Dict1 : CarMaker4SL/Write CM Dict  xname=VC.Gas  xsync=off
  wires:
  Constant/1 -> Write CM Dict1/1

== system generic/CarMaker/VehicleControl/CreateBus VhclCtrl/Braking/Front Camera/While Iterator Subsystem3/If Action Subsystem/If Action Subsystem2 ==
  Action Port : ActionPort  ActionPortLabel=if(u1>1)
  Constant : Constant  Commented=on  Value=30
  Constant1 : Constant  Commented=on  Value=5
  Write CM Dict : CarMaker4SL/Write CM Dict  Commented=on  xname=VC.Steer.AngAcc  xsync=off
  Write CM Dict1 : CarMaker4SL/Write CM Dict  Commented=on  xname=VC.Steer.Ang  xsync=off
  wires:
  Constant/1 -> Write CM Dict/1
  Constant1/1 -> Write CM Dict1/1

== system generic/CarMaker/VehicleControl/CreateBus VhclCtrl/Braking/Front Camera/While Iterator Subsystem3/If Action Subsystem/If Action Subsystem4 ==
  Action Port : ActionPort  ActionPortLabel=else

== system generic/CarMaker/VehicleControl/CreateBus VhclCtrl/Braking/Front Camera/While Iterator Subsystem3/If Action Subsystem2/If Action Subsystem1 ==
  Action Port : ActionPort  ActionPortLabel=if(u1 ==1)
  Constant : Constant  Value=0
  Write CM Dict1 : CarMaker4SL/Write CM Dict  xname=VC.Gas  xsync=off
  wires:
  Constant/1 -> Write CM Dict1/1
